simulink model "Iface"  (R2018b)
settings: Solver=FixedStepDiscrete  StartTime=0.0  StopTime=10.0  RelTol=1e-3
settings Model: Creator=matlab  LastModifiedBy=matlab
settings DataIOCC: SaveOutput=off  SignalLogging=off  SaveTime=off
settings OptimizationCC: DefaultParameterBehavior=Inlined  EnhancedBackFolding=on  PassReuseOutputArgsAs=Individual arguments  OptimizeBlockOrder=speed  DifferentSizesBufferReuse=on  OptimizationCustomize=off
settings DebuggingCC: ParameterTunabilityLossMsg=error
settings SFSimCC: MATLABDynamicMemAlloc=off
settings RTWCC: SystemTargetFile=ert.tlc  TemplateMakefile=ert_default_tmf  PostCodeGenCommand=packNGo(buildInfo);  GenerateReport=on  IncludeHyperlinkInReport=on  LaunchReport=on  GenerateTraceInfo=on  GenerateTraceReport=on  GenerateTraceReportSl=on  GenerateTraceReportSf=on  GenerateTraceReportEml=on
settings CodeAppCC: ForceParamTrailComments=on  IgnoreCustomStorageClasses=off  OperatorAnnotations=on  SimulinkDataObjDesc=on  SFDataObjDesc=on  InsertBlockDesc=on
settings ERTTargetCC: TargetLangStandard=C99 (ISO)  GenerateSampleERTMain=on  InlinedParameterPlacement=NonHierarchical  ERTCustomFileTemplate=example_file_process.tlc

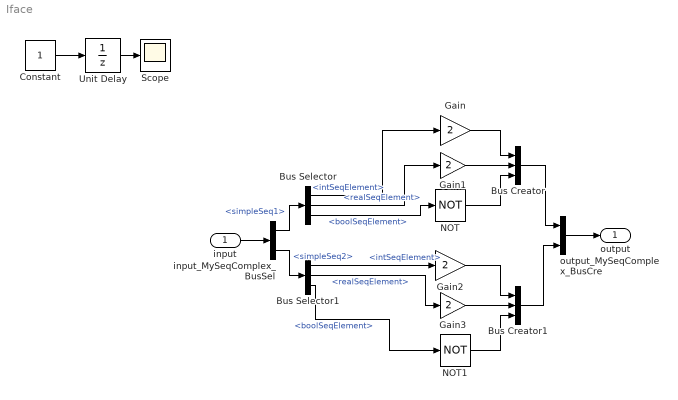
== system Iface ==
  input : Inport  OutDataTypeStr=Bus: MySeqComplex  BusOutputAsStruct=on
  Bus Creator : BusCreator  Inputs=3  OutDataTypeStr=Bus: MySeqSimple  NonVirtualBus=on
      settings: InheritFromInputs=off
  Bus Creator1 : BusCreator  Inputs=3  OutDataTypeStr=Bus: MySeqSimple  NonVirtualBus=on
      settings: InheritFromInputs=off
  Bus Selector : BusSelector  OutputSignals=intSeqElement,realSeqElement,boolSeqElement
  Bus Selector1 : BusSelector  OutputSignals=intSeqElement,realSeqElement,boolSeqElement
  Constant : Constant
  Gain : Gain  Gain=2  OutDataTypeStr=uint16
  Gain1 : Gain  Gain=2  OutDataTypeStr=double
  Gain2 : Gain  Gain=2  OutDataTypeStr=uint16
  Gain3 : Gain  Gain=2  OutDataTypeStr=double
  NOT : Logic  Operator=NOT  IconShape=distinctive  AllPortsSameDT=off  OutDataTypeStr=boolean
  NOT1 : Logic  Operator=NOT  IconShape=distinctive  AllPortsSameDT=off  OutDataTypeStr=boolean
  Scope : Scope
  Unit Delay : UnitDelay  SampleTime=-1
  input_MySeqComplex_BusSel : BusSelector  OutputSignals=simpleSeq1,simpleSeq2
  output_MySeqComplex_BusCre : BusCreator  Inputs=2  OutDataTypeStr=Bus: MySeqComplex  NonVirtualBus=on
      settings: InheritFromInputs=off
  output : Outport  OutDataTypeStr=Bus: MySeqComplex  BusOutputAsStruct=on
  wires:
  input/1 -> input_MySeqComplex_BusSel/1
  output_MySeqComplex_BusCre/1 -> output/1
  Unit Delay/1 -> Scope/1
  Constant/1 -> Unit Delay/1
  input_MySeqComplex_BusSel/1 -> Bus Selector/1  "<simpleSeq1>"
  Bus Selector/1 -> Gain/1  "<intSeqElement>"
  Bus Selector/2 -> Gain1/1  "<realSeqElement>"
  Gain/1 -> Bus Creator/1
  Gain1/1 -> Bus Creator/2
  Bus Creator/1 -> output_MySeqComplex_BusCre/1
  Bus Selector/3 -> NOT/1  "<boolSeqElement>"
  NOT/1 -> Bus Creator/3
  Gain3/1 -> Bus Creator1/2
  Gain2/1 -> Bus Creator1/1
  NOT1/1 -> Bus Creator1/3
  input_MySeqComplex_BusSel/2 -> Bus Selector1/1  "<simpleSeq2>"
  Bus Selector1/1 -> Gain2/1  "<intSeqElement>"
  Bus Selector1/3 -> NOT1/1  "<boolSeqElement>"
  Bus Selector1/2 -> Gain3/1  "<realSeqElement>"
  Bus Creator1/1 -> output_MySeqComplex_BusCre/2
